simulink model "SVPWM_self"  (R2022a)
settings: Solver=FixedStepAuto  StartTime=0.0  StopTime=stoptime  FixedStep=stepsize  MaxStep=2e-6  RelTol=1e-3
undefined symbols (not defined in the file or in its folder): Continuous, frequency, fs, gcbh, L, R, sps, sps_rtmsupport, spsSawtoothGeneratorModel, stepsize, u_sampletime, V, Vdc
libraries: spsIGBTDiodeLib x6, spsVoltageMeasurementLib x5, spsSeriesRLCBranchLib x4, spsParallelRLCBranchLib x2, spsGroundLib x1, spsThreePhaseVIMeasurementLib x1, spsDCVoltageSourceLib x1, simulink_extras x1, eeTransforms x1, spspowerguiLib x1
settings Model: Creator=Bob  LastModifiedBy=Bob

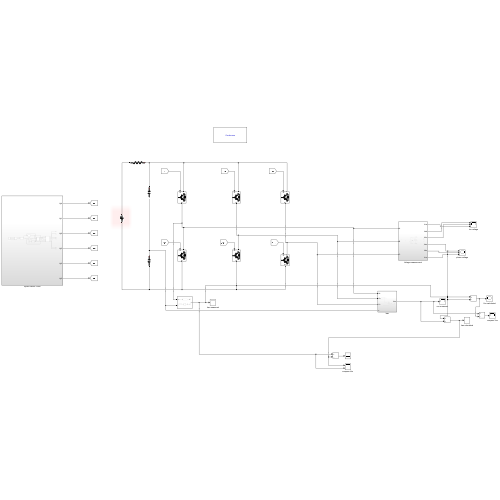
[thumbnail: Simulink's stored preview of the top-level diagram]
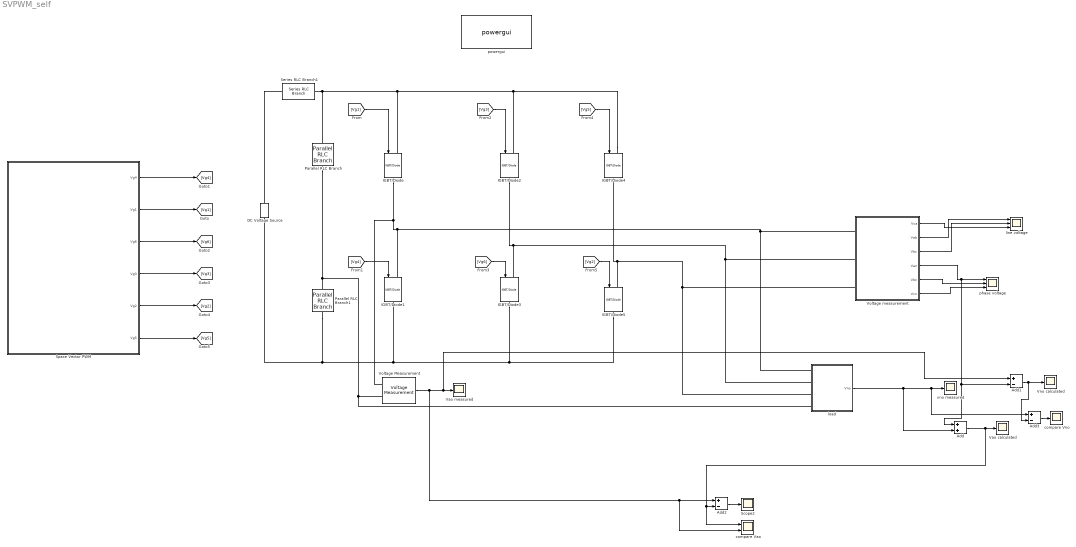
== system SVPWM_self ==
  " load" : Subsystem
  Add : Sum
  Add1 : Sum  Inputs=+-
  Add2 : Sum  Inputs=+-
  Add3 : Sum  Inputs=+-
  DC Voltage Source : spsDCVoltageSourceLib/DC Voltage Source  Amplitude=Vdc  Measurements=None
  IGBT/Diode{,1..5} (6 alike) : spsIGBTDiodeLib/IGBT//Diode  Ron=1e-3  Rs=1e5  Cs=inf  Measurements=off
  Parallel RLC Branch : spsParallelRLCBranchLib/Parallel RLC Branch  LConnTagsString=a  RConnTagsString=__new0  BranchType=C  Resistance=1  Inductance=1e-3  SetiL0=off  InitialCurrent=0  Capacitance=470e-4  Setx0=off  InitialVoltage=1  Measurements=None
  Parallel RLC Branch1 : spsParallelRLCBranchLib/Parallel RLC Branch  LConnTagsString=a  RConnTagsString=__new0  BranchType=C  Resistance=1  Inductance=1e-3  SetiL0=off  InitialCurrent=0  Capacitance=470e-4  Setx0=off  InitialVoltage=1  Measurements=None
  Scope2 : Scope
  Series RLC Branch1 : spsSeriesRLCBranchLib/Series RLC Branch  LConnTagsString=__new0  RConnTagsString=__new0  BranchType=R  Resistance=0.001  Inductance=100e-3  SetiL0=off  InitialCurrent=0  Capacitance=1e-6  Setx0=off  InitialVoltage=0  Measurements=None
  Space Vector PWM : Subsystem
  Vao calculated : Scope
  Vao measured : Scope
  Vno calculated : Scope
  Voltage Measurement : spsVoltageMeasurementLib/Voltage Measurement  PhasorSimulation=off  OutputType=Complex  PSBequivalent=0
  "Voltage measurement " : Subsystem
  compare Vao : Scope  NumInputPorts=2
  compare Vno : Scope
  line voltage : Scope  NumInputPorts=3
  phase voltage : Scope  NumInputPorts=3
  powergui : spspowerguiLib/powergui  Priority=1  SimulationMode=Continuous  SampleTime=stepsize  frequency=60  Iterations=50  frequencyindice=0  Pbase=100e6  ErrMax=1e-4  UnitsV=kV  UnitsW=MW  buscounter=0  FunctionMessages=off  echomessages=off  EnableUseOfTLC=off  CurrentSourceSwitches=off  DisableSnubberDevices=off  DisableRonSwitches=off  DisableVfSwitches=off  DisplayEquations=off  AutomaticDiscreteSolvers=off  SolverType=Tustin/Backward Euler (TBE)  Interpol=off  ExternalGateDelay=off  methode=off  Ts=100  x0status=blocks  SPID=on  SwTol=0  HookPort=off  NonlinearTolerance=1e-4  nMaxIteration=100  ContinueOnMaxIteration=off  RestoreLinks=warning  ResistiveCurrentMeasurement=off  Frange=[0:2:500]  Ylog=off  Xlog=on  ShowGrid=off  save=off  variable=ZData  structure=0  ZoomFFT=off  StartTime=0.0  cycles=1  DisplayStyle=1  fundamental=60  FreqAxis=off  MaxFrequency=1000  frequencyindicesteady=1  RmsSteady=1  display=off
  vno measured : Scope
  wires:
  Space Vector PWM/2(Vg1) -> [Vg1]
  Space Vector PWM/1(Vg4) -> [Vg4]
  Space Vector PWM/3(Vg6) -> [Vg6]
  Space Vector PWM/4(Vg3) -> [Vg3]
  Space Vector PWM/5(Vg2) -> [Vg2]
  Space Vector PWM/6(Vg5) -> [Vg5]
  [Vg6] -> IGBT/Diode3/1
  [Vg2] -> IGBT/Diode5/1
  [Vg3] -> IGBT/Diode2/1
  [Vg4] -> IGBT/Diode1/1
  "Voltage measurement "/1(Vca) -> line voltage/3
  "Voltage measurement "/2(Vab) -> line voltage/1
  "Voltage measurement "/3(Vbc) -> line voltage/2
  "Voltage measurement "/4(Van) -> Add1/2, Add/1, phase voltage/1
  "Voltage measurement "/5(Vbn) -> phase voltage/2
  "Voltage measurement "/6(Vcn) -> phase voltage/3
  [Vg1] -> IGBT/Diode/1
  [Vg5] -> IGBT/Diode4/1
  Voltage Measurement/1 -> compare Vao/2, Add2/1, Add1/1, Vao measured/1
  " load"/1(Vno) -> Add/2, vno measured/1, Add3/1
  Add/1 -> compare Vao/1, Add2/2, Vao calculated/1
  Add1/1 -> Add3/2, Vno calculated/1
  Add2/1 -> Scope2/1
  Add3/1 -> compare Vno/1
  connections:
  IGBT/Diode4/LConn1 -- Parallel RLC Branch/LConn1 -- Series RLC Branch1/LConn1 -- IGBT/Diode/LConn1 -- IGBT/Diode2/LConn1
  IGBT/Diode3/RConn1 -- IGBT/Diode5/RConn1 -- IGBT/Diode1/RConn1 -- Parallel RLC Branch1/RConn1 -- DC Voltage Source/LConn1
  " load"/LConn2 -- "Voltage measurement "/LConn2 -- IGBT/Diode3/LConn1 -- IGBT/Diode2/RConn1
  " load"/LConn1 -- "Voltage measurement "/LConn1 -- IGBT/Diode1/LConn1 -- IGBT/Diode/RConn1 -- Voltage Measurement/LConn1
  " load"/LConn3 -- "Voltage measurement "/LConn3 -- IGBT/Diode4/RConn1 -- IGBT/Diode5/LConn1
  DC Voltage Source/RConn1 -- Series RLC Branch1/RConn1
  Parallel RLC Branch/RConn1 -- " load"/LConn4 -- Voltage Measurement/LConn2 -- Parallel RLC Branch1/LConn1

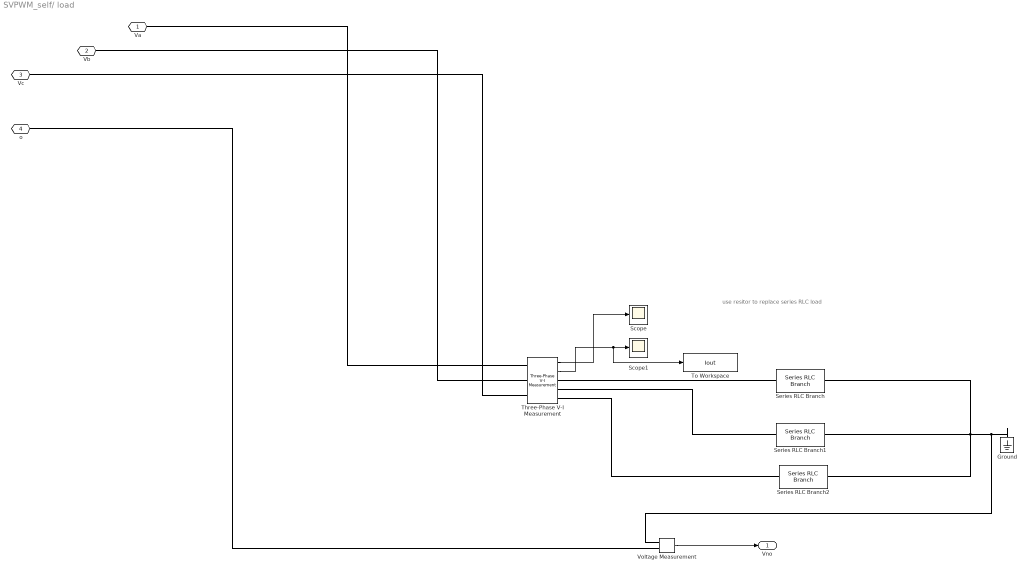
== system SVPWM_self/ load ==
  note: use resitor to replace series RLC load
  Ground : spsGroundLib/Ground  LConnTagsString=a
  Scope : Scope
  Scope1 : Scope
  Series RLC Branch : spsSeriesRLCBranchLib/Series RLC Branch  LConnTagsString=__new0  RConnTagsString=__new0  BranchType=RL  Resistance=R  Inductance=L  SetiL0=off  InitialCurrent=0  Capacitance=1e-6  Setx0=off  InitialVoltage=0  Measurements=None
  Series RLC Branch1 : spsSeriesRLCBranchLib/Series RLC Branch  LConnTagsString=__new0  RConnTagsString=__new0  BranchType=RL  Resistance=R  Inductance=L  SetiL0=off  InitialCurrent=0  Capacitance=1e-6  Setx0=off  InitialVoltage=0  Measurements=None
  Series RLC Branch2 : spsSeriesRLCBranchLib/Series RLC Branch  LConnTagsString=__new0  RConnTagsString=__new0  BranchType=RL  Resistance=R  Inductance=L  SetiL0=off  InitialCurrent=0  Capacitance=1e-6  Setx0=off  InitialVoltage=0  Measurements=None
  Three-Phase V-I Measurement : spsThreePhaseVIMeasurementLib/Three-Phase V-I Measurement  VoltageMeasurement=phase-to-ground  SetLabelV=off  LabelV=Vabc  Vpu=off  VpuLL=off  CurrentMeasurement=yes  SetLabelI=off  LabelI=Iabc  Ipu=off  Pbase=100e6  Vbase=500e3  OutputType=Complex  PhasorSimulation=off  PSBequivalent=0
  To Workspace : ToWorkspace  VariableName=Iout  SampleTime=-1
      settings: Save2DSignal=2-D array (concatenate along first dimension)
  Voltage Measurement : spsVoltageMeasurementLib/Voltage Measurement  PhasorSimulation=off  OutputType=Complex  PSBequivalent=0
  Va : PMIOPort  Side=Left
  Vb : PMIOPort  Port=2  Side=Left
  Vc : PMIOPort  Port=3  Side=Left
  o : PMIOPort  Port=4  Side=Left
  Vno : Outport
  wires:
  Three-Phase V-I Measurement/2 -> To Workspace/1, Scope1/1
  Three-Phase V-I Measurement/1 -> Scope/1
  Voltage Measurement/1 -> Vno/1
  connections:
  Three-Phase V-I Measurement/LConn2 -- Vb/RConn1
  Three-Phase V-I Measurement/LConn3 -- Vc/RConn1
  Three-Phase V-I Measurement/LConn1 -- Va/RConn1
  Ground/LConn1 -- Voltage Measurement/LConn1 -- Series RLC Branch2/RConn1 -- Series RLC Branch1/RConn1 -- Series RLC Branch/RConn1
  Series RLC Branch/LConn1 -- Three-Phase V-I Measurement/RConn1
  Series RLC Branch1/LConn1 -- Three-Phase V-I Measurement/RConn2
  Series RLC Branch2/LConn1 -- Three-Phase V-I Measurement/RConn3
  Voltage Measurement/LConn2 -- o/RConn1

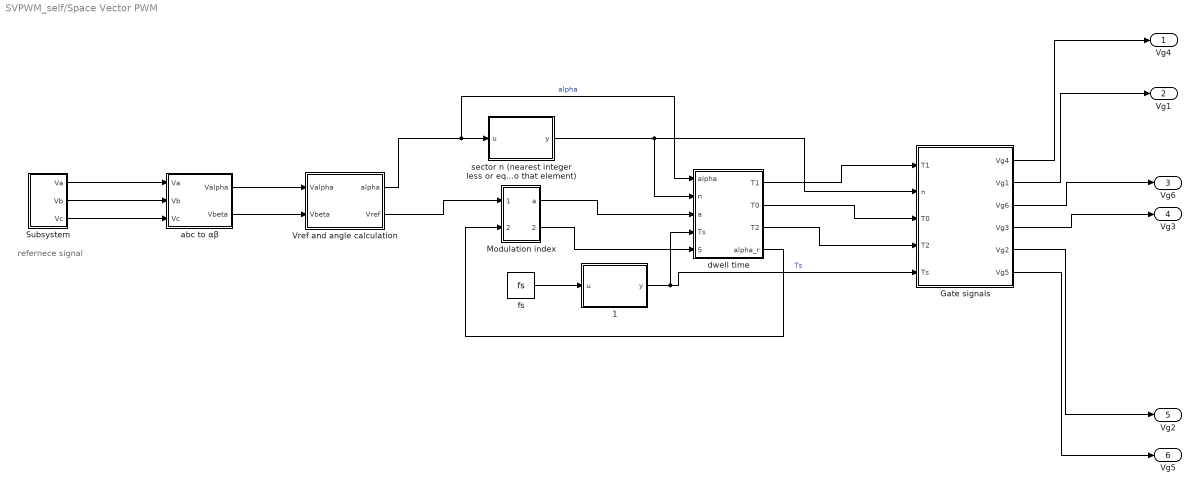
== system SVPWM_self/Space Vector PWM ==
  note: refernece signal
  1 : MATLAB Function  TreatAsAtomicUnit=on
  Gate signals : Subsystem
  Modulation index : Subsystem
  Subsystem : Subsystem
  Vref and angle calculation : Subsystem
  abc to αβ : Subsystem
  "dwell time " : Subsystem
  fs : Constant  Value=fs
  sector n (nearest integer less or equal to that element) : MATLAB Function  TreatAsAtomicUnit=on
  Vg4 : Outport
  Vg1 : Outport  Port=2
  Vg6 : Outport  Port=3
  Vg3 : Outport  Port=4
  Vg2 : Outport  Port=5
  Vg5 : Outport  Port=6
  wires:
  "dwell time "/1(T1) -> Gate signals/1(T1)
  Subsystem/2(Vb) -> abc to αβ/2(Vb)
  Subsystem/3(Vc) -> abc to αβ/3(Vc)
  Vref and angle calculation/1(alpha) -> "dwell time "/1(alpha), sector n (nearest integer less or equal to that element)/1(u)  "alpha"
  abc to αβ/1(Valpha) -> Vref and angle calculation/1(Valpha)
  abc to αβ/2(Vbeta) -> Vref and angle calculation/2(Vbeta)
  Subsystem/1(Va) -> abc to αβ/1(Va)
  Gate signals/2(Vg1) -> Vg1/1
  Vref and angle calculation/2(Vref) -> Modulation index/1(Vref)
  sector n (nearest integer less or equal to that element)/1(y) -> "dwell time "/2(n), Gate signals/2(n)
  "dwell time "/3(T2) -> Gate signals/4(T2)
  Gate signals/5(Vg2) -> Vg2/1
  "dwell time "/2(T0) -> Gate signals/3(T0)
  Gate signals/4(Vg3) -> Vg3/1
  Gate signals/1(Vg4) -> Vg4/1
  Gate signals/3(Vg6) -> Vg6/1
  Gate signals/6(Vg5) -> Vg5/1
  Modulation index/1(a) -> "dwell time "/3(a)
  fs/1 -> 1/1(u)
  1/1(y) -> Gate signals/5(Ts), "dwell time "/4(Ts)  "Ts"
  "dwell time "/4(alpha_r) -> Modulation index/2(alpha_r)
  Modulation index/2(Outport) -> "dwell time "/5(alpha_m)

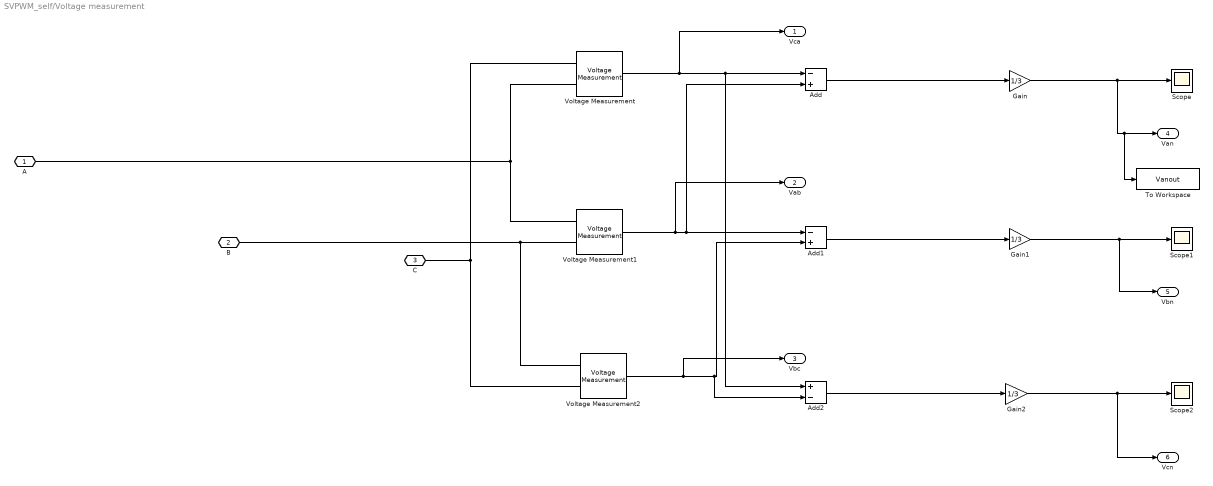
== system SVPWM_self/Voltage measurement  ==
  Add : Sum  Inputs=-+
  Add1 : Sum  Inputs=-+
  Add2 : Sum  Inputs=+-
  Gain : Gain  Gain=1/3
  Gain1 : Gain  Gain=1/3
  Gain2 : Gain  Gain=1/3
  Scope : Scope
  Scope1 : Scope
  Scope2 : Scope
  To Workspace : ToWorkspace  VariableName=Vanout  SampleTime=-1
      settings: Save2DSignal=2-D array (concatenate along first dimension)
  Voltage Measurement : spsVoltageMeasurementLib/Voltage Measurement  PhasorSimulation=off  OutputType=Complex  PSBequivalent=0
  Voltage Measurement1 : spsVoltageMeasurementLib/Voltage Measurement  PhasorSimulation=off  OutputType=Complex  PSBequivalent=0
  Voltage Measurement2 : spsVoltageMeasurementLib/Voltage Measurement  PhasorSimulation=off  OutputType=Complex  PSBequivalent=0
  A : PMIOPort  Side=Left
  B : PMIOPort  Port=2  Side=Left
  C : PMIOPort  Port=3  Side=Left
  Vca : Outport
  Vab : Outport  Port=2
  Vbc : Outport  Port=3
  Van : Outport  Port=4
  Vbn : Outport  Port=5
  Vcn : Outport  Port=6
  wires:
  Gain2/1 -> Vcn/1, Scope2/1
  Gain/1 -> To Workspace/1, Van/1, Scope/1
  Voltage Measurement1/1 -> Vab/1, Add/2, Add1/1
  Voltage Measurement2/1 -> Vbc/1, Add2/2, Add1/2
  Gain1/1 -> Vbn/1, Scope1/1
  Add/1 -> Gain/1
  Add1/1 -> Gain1/1
  Voltage Measurement/1 -> Vca/1, Add2/1, Add/1
  Add2/1 -> Gain2/1
  connections:
  Voltage Measurement/LConn2 -- Voltage Measurement1/LConn1 -- A/RConn1
  Voltage Measurement1/LConn2 -- B/RConn1 -- Voltage Measurement2/LConn1
  Voltage Measurement2/LConn2 -- Voltage Measurement/LConn1 -- C/RConn1

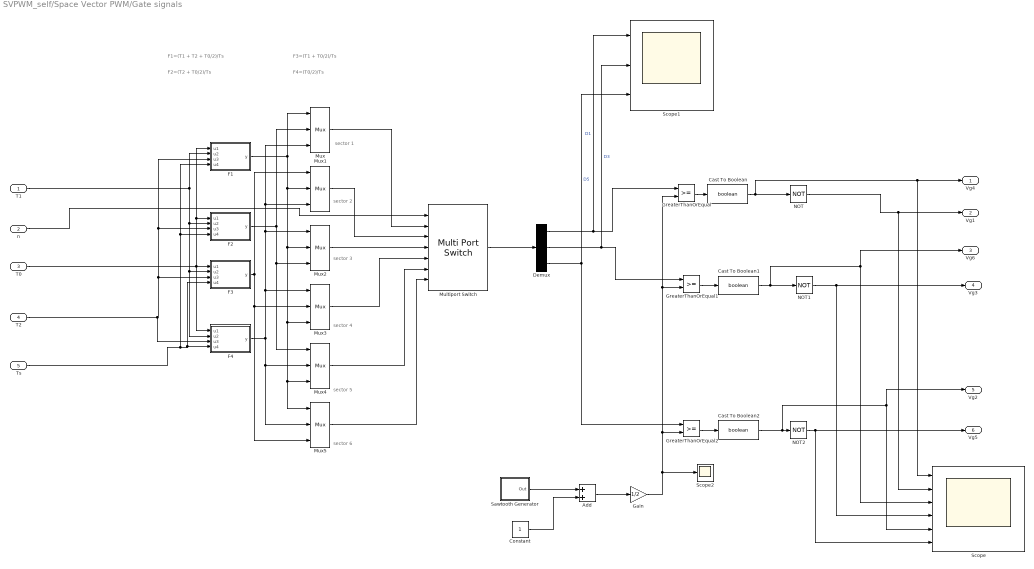
== system SVPWM_self/Space Vector PWM/Gate signals ==
  note: F4=(T0/2)/Ts
  note: F3=(T1 + T0/2)/Ts
  note: F2=(T2 + T0/2)/Ts
  note: F1=(T1 + T2 + T0/2)/Ts
  note: sector 2
  note: sector 3
  note: sector 4
  note: sector 5
  note: sector 6
  note: sector 1
  T1 : Inport
  n : Inport  Port=2
  T0 : Inport  Port=3
  T2 : Inport  Port=4
  Ts : Inport  Port=5
  Add : Sum
  Cast To Boolean : DataTypeConversion  OutDataTypeStr=boolean  SaturateOnIntegerOverflow=off  RndMeth=Floor
  Cast To Boolean1 : DataTypeConversion  OutDataTypeStr=boolean  SaturateOnIntegerOverflow=off  RndMeth=Floor
  Cast To Boolean2 : DataTypeConversion  OutDataTypeStr=boolean  SaturateOnIntegerOverflow=off  RndMeth=Floor
  Constant : Constant
  Demux : Demux  Outputs=3
  F1 : MATLAB Function  TreatAsAtomicUnit=on
  F2 : MATLAB Function  TreatAsAtomicUnit=on
  F3 : MATLAB Function  TreatAsAtomicUnit=on
  F4 : MATLAB Function  TreatAsAtomicUnit=on
  Gain : Gain  Gain=1/2
  GreaterThanOrEqual : RelationalOperator  OutDataTypeStr=boolean  RndMeth=Simplest  InputSameDT=off
  GreaterThanOrEqual1 : RelationalOperator  OutDataTypeStr=boolean  RndMeth=Simplest  InputSameDT=off
  GreaterThanOrEqual2 : RelationalOperator  OutDataTypeStr=boolean  RndMeth=Simplest  InputSameDT=off
  Multiport Switch : MultiPortSwitch  Inputs=6  DiagnosticForDefault=None  SaturateOnIntegerOverflow=off  InputSameDT=off
  Mux{,1..5} (6 alike) : Mux  Inputs=3
  NOT : Logic  Operator=NOT  IconShape=distinctive  AllPortsSameDT=off  OutDataTypeStr=boolean
  NOT1 : Logic  Operator=NOT  IconShape=distinctive  AllPortsSameDT=off  OutDataTypeStr=boolean
  NOT2 : Logic  Operator=NOT  IconShape=distinctive  AllPortsSameDT=off  OutDataTypeStr=boolean
  Sawtooth Generator : Subsystem  AncestorBlock=spsSawtoothGeneratorLib/Sawtooth Generator  DialogController=POWERSYS.PowerSysDialog  LoadFcn=sps_rtmsupport('LoadFcn', gcbh);  StartFcn=sps_rtmsupport('StartFcn', gcbh);  StopFcn=sps_rtmsupport('StopFcn', gcbh);  mask(Sawtooth Generator){Freq=fs, Phase=0, Ts=0}
      mask prompts: Freq "Frequency (Hz):"; Phase "Phase (degrees):"; Ts "Sample time:"
      mask help: Generate a sawtooth wave with peak of -1 to +1.
      mask init:
      | block = gcb;
      | [WantBlockChoice,Ts,sps] = powericon('SawtoothGeneratorInit',block,Phase,Freq,Ts);
      | powericon('SetInternalModels','set',block,WantBlockChoice);
      settings: CopyFcn=sps_rtmsupport('CopyFcn', gcbh);  DeleteFcn=sps_rtmsupport('DeleteFcn', gcbh);  UndoDeleteFcn=sps_rtmsupport('UndoDeleteFcn', gcbh);  ModelCloseFcn=sps_rtmsupport('ModelCloseFcn', gcbh);  PreSaveFcn=sps_rtmsupport('PreSaveFcn', gcbh);  PostSaveFcn=sps_rtmsupport('PostSaveFcn', gcbh);  NameChangeFcn=sps_rtmsupport('NameChangeFcn', gcbh);  PreCopyFcn=sps_rtmsupport('PreCopyFcn', gcbh);  OpenFcn=sps_rtmsupport('OpenFcn', gcbh, []);  CloseFcn=sps_rtmsupport('CloseFcn', gcbh);  PreDeleteFcn=sps_rtmsupport('PreDeleteFcn', gcbh);
      mask Help: helpview(psbhelp);
      mask Display: plot([sps.time sps.time+sps.time(end)],repmat(sps.Out,1,2))
  Scope : Scope  NumInputPorts=6
  Scope1 : Scope  NumInputPorts=3
  Scope2 : Scope
  Vg4 : Outport
  Vg1 : Outport  Port=2
  Vg6 : Outport  Port=3
  Vg3 : Outport  Port=4
  Vg2 : Outport  Port=5
  Vg5 : Outport  Port=6
  wires:
  T0/1 -> F4/1(u1), F1/1(u1), F2/1(u1), F3/1(u1)
  Demux/2 -> Scope1/2, GreaterThanOrEqual1/1  "D3"
  T1/1 -> F4/2(u2), F3/2(u2), F2/2(u2), F1/2(u2)
  n/1 -> Multiport Switch/1
  Gain/1 -> Scope2/1, GreaterThanOrEqual2/2, GreaterThanOrEqual/2, GreaterThanOrEqual1/2
  F1/1(y) -> Mux5/1, Mux4/3, Mux3/3, Mux2/2, Mux1/2, Mux/1
  F4/1(y) -> Mux3/1, Mux2/1, Mux1/3, Mux/3, Mux5/2, Mux4/2
  GreaterThanOrEqual1/1 -> Cast To Boolean1/1
  Mux1/1 -> Multiport Switch/3
  Mux2/1 -> Multiport Switch/4
  NOT1/1 -> Vg3/1, Scope/4
  NOT2/1 -> Vg5/1, Scope/6
  GreaterThanOrEqual/1 -> Cast To Boolean/1
  T2/1 -> F4/3(u3), F3/3(u3), F2/3(u3), F1/3(u3)
  Mux/1 -> Multiport Switch/2
  GreaterThanOrEqual2/1 -> Cast To Boolean2/1
  NOT/1 -> Vg1/1, Scope/2
  Ts/1 -> F1/4(u4), F2/4(u4), F3/4(u4), F4/4(u4)
  Demux/1 -> Scope1/1, GreaterThanOrEqual/1  "D1"
  Demux/3 -> GreaterThanOrEqual2/1, Scope1/3  "D5"
  F3/1(y) -> Mux1/1, Mux5/3, Mux3/2
  Mux5/1 -> Multiport Switch/7
  Mux3/1 -> Multiport Switch/5
  F2/1(y) -> Mux4/1, Mux2/3, Mux/2
  Sawtooth Generator/1(Out) -> Add/1
  Multiport Switch/1 -> Demux/1
  Mux4/1 -> Multiport Switch/6
  Add/1 -> Gain/1
  Constant/1 -> Add/2
  Cast To Boolean/1 -> Vg4/1, Scope/1, NOT/1
  Cast To Boolean1/1 -> Vg6/1, Scope/3, NOT1/1
  Cast To Boolean2/1 -> Vg2/1, Scope/5, NOT2/1

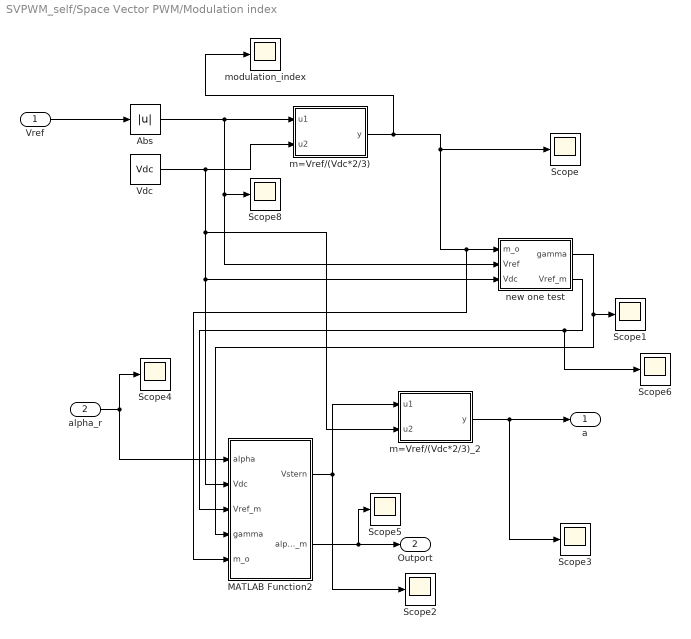
== system SVPWM_self/Space Vector PWM/Modulation index ==
  Vref : Inport
  alpha_r : Inport  Port=2
  Abs : Abs  SaturateOnIntegerOverflow=off
  MATLAB Function2 : MATLAB Function  TreatAsAtomicUnit=on
  Scope{,1..6,8} (8 alike) : Scope
  Vdc : Constant  Value=Vdc
  m=Vref/(Vdc*2/3) : MATLAB Function  TreatAsAtomicUnit=on
  m=Vref/(Vdc*2/3)_2 : MATLAB Function  TreatAsAtomicUnit=on
  modulation_index : Scope
  new one test : MATLAB Function  TreatAsAtomicUnit=on
  a : Outport
  Outport : Outport  Port=2
  wires:
  Abs/1 -> new one test/2(Vref), Scope8/1, m=Vref/(Vdc*2/3)/1(u1)
  m=Vref/(Vdc*2/3)/1(y) -> MATLAB Function2/5(m_o), new one test/1(m_o), Scope/1, modulation_index/1
  Vref/1 -> Abs/1
  Vdc/1 -> m=Vref/(Vdc*2/3)/2(u2), new one test/3(Vdc), MATLAB Function2/2(Vdc), m=Vref/(Vdc*2/3)_2/2(u2)
  alpha_r/1 -> MATLAB Function2/1(alpha), Scope4/1
  MATLAB Function2/1(Vstern) -> Scope2/1, m=Vref/(Vdc*2/3)_2/1(u1)
  m=Vref/(Vdc*2/3)_2/1(y) -> Scope3/1, a/1
  new one test/1(gamma) -> Scope1/1, MATLAB Function2/4(gamma)
  MATLAB Function2/2(alpha_m) -> Scope5/1, Outport/1
  new one test/2(Vref_m) -> Scope6/1, MATLAB Function2/3(Vref_m)

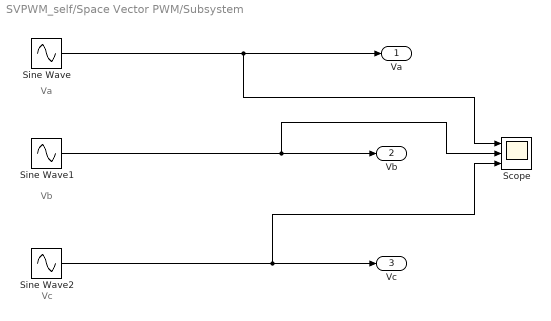
== system SVPWM_self/Space Vector PWM/Subsystem ==
  note: Va
  note: Vb
  note: Vc
  Scope : Scope  NumInputPorts=3
  Sine Wave : Sin  Amplitude=V  Frequency=2*pi*frequency  SampleTime=0
  Sine Wave1 : Sin  Amplitude=V  Frequency=2*pi*frequency  Phase=-2*pi/3  SampleTime=0
  Sine Wave2 : Sin  Amplitude=V  Frequency=2*pi*frequency  Phase=-4*pi/3  SampleTime=0
  Va : Outport
  Vb : Outport  Port=2
  Vc : Outport  Port=3
  wires:
  Sine Wave1/1 -> Vb/1, Scope/2
  Sine Wave2/1 -> Vc/1, Scope/3
  Sine Wave/1 -> Va/1, Scope/1

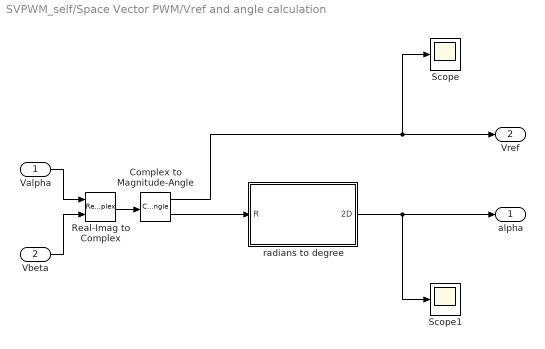
== system SVPWM_self/Space Vector PWM/Vref and angle calculation ==
  Valpha : Inport
  Vbeta : Inport  Port=2
  Complex to Magnitude-Angle : ComplexToMagnitudeAngle
  Real-Imag to Complex : RealImagToComplex
  Scope : Scope
  Scope1 : Scope
  radians to degree : Subsystem
  alpha : Outport
  Vref : Outport  Port=2
  wires:
  Complex to Magnitude-Angle/2 -> radians to degree/1(R)
  Complex to Magnitude-Angle/1 -> Scope/1, Vref/1
  Valpha/1 -> Real-Imag to Complex/1
  Vbeta/1 -> Real-Imag to Complex/2
  radians to degree/1(2D) -> Scope1/1, alpha/1
  Real-Imag to Complex/1 -> Complex to Magnitude-Angle/1

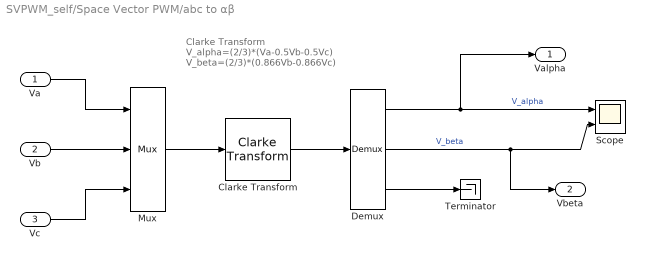
== system SVPWM_self/Space Vector PWM/abc to αβ ==
  note: Clarke Transform
      | V_alpha=(2/3)*(Va-0.5Vb-0.5Vc)
      | V_beta=(2/3)*(0.866Vb-0.866Vc)
  Va : Inport
  Vb : Inport  Port=2
  Vc : Inport  Port=3
  Clarke Transform : eeTransforms/Clarke Transform  PowerInvariant=off
      settings: SourceProductBaseCode=PS
  Demux : Demux  Outputs=3
  Mux : Mux  Inputs=3
  Scope : Scope  NumInputPorts=2
  Terminator : Terminator
  Valpha : Outport
  Vbeta : Outport  Port=2
  wires:
  Demux/2 -> Vbeta/1, Scope/2  "V_beta"
  Clarke Transform/1 -> Demux/1
  Demux/3 -> Terminator/1
  Demux/1 -> Valpha/1, Scope/1  "V_alpha"
  Va/1 -> Mux/1
  Vb/1 -> Mux/2
  Vc/1 -> Mux/3
  Mux/1 -> Clarke Transform/1

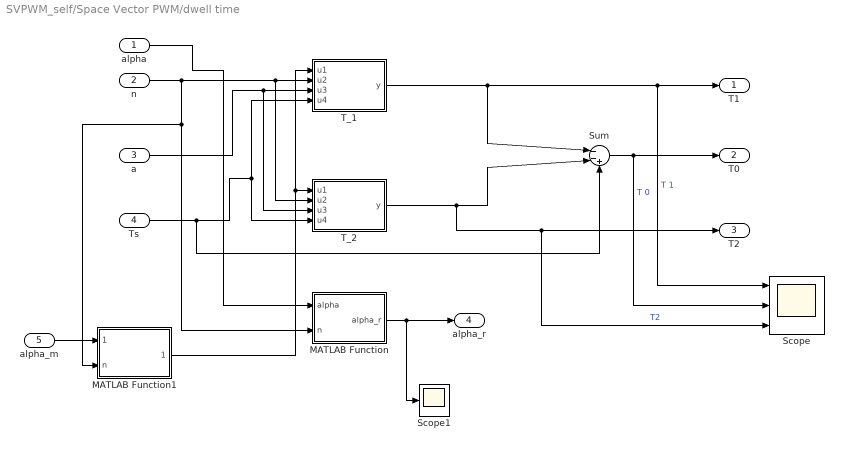
== system SVPWM_self/Space Vector PWM/dwell time  ==
  alpha : Inport
  n : Inport  Port=2
  a : Inport  Port=3
  Ts : Inport  Port=4
  alpha_m : Inport  Port=5
  MATLAB Function : MATLAB Function  TreatAsAtomicUnit=on
  MATLAB Function1 : MATLAB Function  TreatAsAtomicUnit=on
  Scope : Scope  NumInputPorts=3
  Scope1 : Scope
  Sum : Sum  Inputs=|--+
  T_1 : MATLAB Function  TreatAsAtomicUnit=on
  T_2 : MATLAB Function  TreatAsAtomicUnit=on
  T1 : Outport
  T0 : Outport  Port=2
  T2 : Outport  Port=3
  alpha_r : Outport  Port=4
  wires:
  T_1/1(y) -> Scope/1, T1/1, Sum/1  "T 1"
  T_2/1(y) -> Scope/3, T2/1, Sum/2  "T2"
  alpha/1 -> MATLAB Function/1(alpha)
  n/1 -> MATLAB Function1/2(n), MATLAB Function/2(n), T_2/2(u2), T_1/2(u2)
  a/1 -> T_2/3(u3), T_1/3(u3)
  Ts/1 -> Sum/3, T_1/4(u4), T_2/4(u4)
  Sum/1 -> Scope/2, T0/1  "T 0"
  MATLAB Function/1(alpha_r) -> Scope1/1, alpha_r/1
  alpha_m/1 -> MATLAB Function1/1(alpha_m)
  MATLAB Function1/1(alpha_mr) -> T_2/1(u1), T_1/1(u1)

== system SVPWM_self/Space Vector PWM/Gate signals/Sawtooth Generator ==
  Model : Subsystem  AncestorBlock=spsSawtoothGeneratorModel/Continuous
  Out : Outport  VectorParamsAs1DForOutWhenUnconnected=off
  wires:
  Model/1(Out) -> Out/1

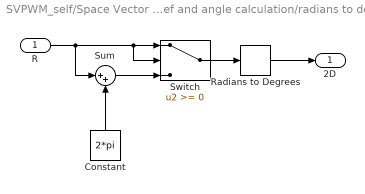
== system SVPWM_self/Space Vector PWM/Vref and angle calculation/radians to degree ==
  R : Inport
  Constant : Constant  Value=2*pi
  Radians to Degrees : simulink_extras/Transformations/Radians to Degrees
  Sum : Sum  Inputs=|++
  Switch : Switch  SaturateOnIntegerOverflow=off  InputSameDT=off
  2D : Outport
  wires:
  Radians to Degrees/1 -> 2D/1
  Constant/1 -> Sum/2
  R/1 -> Sum/1, Switch/2, Switch/1
  Sum/1 -> Switch/3
  Switch/1 -> Radians to Degrees/1

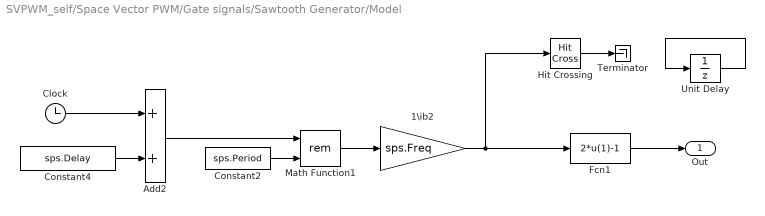
== system SVPWM_self/Space Vector PWM/Gate signals/Sawtooth Generator/Model ==
  1\ib2 : Gain  Gain=sps.Freq  SaturateOnIntegerOverflow=on  OutDataTypeStr=Inherit: Same as input  ParamDataTypeStr=Inherit: Same as input
  Add2 : Sum
  Clock : Clock
  Constant2 : Constant  Value=sps.Period  SampleTime=0
  Constant4 : Constant  Value=sps.Delay  SampleTime=0
  Fcn1 : Fcn  Expr=2*u(1)-1
  Hit Crossing : HitCross
  Math Function1 : Math  Operator=rem  SignedPower=on
  Terminator : Terminator
  Unit Delay : UnitDelay  SampleTime=u_sampletime  HasFrameUpgradeWarning=on
  Out : Outport
  wires:
  Math Function1/1 -> 1\ib2/1
  Clock/1 -> Add2/1
  Constant2/1 -> Math Function1/2
  Constant4/1 -> Add2/2
  Add2/1 -> Math Function1/1
  Unit Delay/1 -> Unit Delay/1
  Fcn1/1 -> Out/1
  1\ib2/1 -> Hit Crossing/1, Fcn1/1
  Hit Crossing/1 -> Terminator/1

== matlab function SVPWM_self/Space Vector PWM/dwell time /MATLAB Function1 ==
  data: alpha_m input; alpha_mr output; n input
function alpha_mr = fcn(alpha_m,n)
alpha_mr=(alpha_m*180/pi+((n-1)*(60)));

== matlab function SVPWM_self/Space Vector PWM/Modulation index/m=Vref//(Vdc*2//3)_2 ==
  data: u1 input; y output; u2 input
function y = fcn(u1,u2)

y = u1/((2/3)*u2);

== matlab function SVPWM_self/Space Vector PWM/Modulation index/MATLAB Function2 ==
  data: alpha input; Vstern output; Vdc input; Vref_m input; gamma input; m_o input; alpha_m output
function [Vstern,alpha_m] = fcn(alpha,Vdc,Vref_m,gamma,m_o)
Vstern=0;
alpha_m=pi;
if gamma==pi/2
    Vstern=Vref_m;
    alpha_m=alpha;
end
if gamma~=pi/2
    if ((m_o>(sqrt(3)/2))&&(m_o<0.9068))
        if ((0<=alpha)&&(alpha<(gamma)))
            Vstern=Vref_m;
            alpha_m=alpha;
        end
        if ((alpha>=(gamma))&&(alpha<((pi/3)-gamma)))
            if (alpha<=(pi/6))
                Vstern=(1/sqrt(3))*Vdc/(cos((pi/6)-alpha)) ;
                alpha_m=alpha;
            end
            if (alpha>(pi/6))
                Vstern=(1/sqrt(3))*Vdc/(cos(alpha-(pi/6))) ;
                alpha_m=alpha;
            end
        end
        if ((((pi/3)-gamma)<=alpha)&&(alpha<(pi/3)))
            Vstern=Vref_m;
            alpha_m=alpha;
        end
    end
    if ((m_o>=0.9068)&&(m_o<0.9517))
        if ((0<=alpha)&&(alpha<(gamma)))
            Vstern=(1/sqrt(3))*Vdc/(cos((pi/6)-alpha));
            alpha_m=alpha;
        end
        if ((alpha>=(gamma))&&(alpha<((pi/3)-gamma)))
            if (alpha<=(pi/6))
                Vstern=(1/sqrt(3))*Vdc/(cos((pi/6)-alpha)) ;
                alpha_m=alpha;
            end
            if (alpha>(pi/6))
                Vstern=(1/sqrt(3))*Vdc/(cos(alpha-(pi/6))) ;
                alpha_m=alpha;
            end
        end
        if ((((pi/3)-gamma)<=alpha)&&(alpha<(pi/3)))
            Vstern=(1/sqrt(3))*Vdc/(cos(alpha-(pi/6))) ;
            alpha_m=alpha;
        end
    end
    if (m_o>=0.9517)
        if ((0<=alpha)&&(alpha<(gamma)))
            Vstern=2*Vdc/3;
            alpha_m=0;
        end
        if ((alpha>=(gamma))&&(alpha<((pi/3)-gamma)))
            if (alpha<=(pi/6))
                Vstern=(1/sqrt(3))*Vdc/(cos((pi/6)-alpha)) ;
                alpha_m=(pi/6)*(alpha-gamma)/((pi/6)-gamma);
            end
            if (alpha>(pi/6))
                Vstern=(1/sqrt(3))*Vdc/(cos(alpha-(pi/6))) ;
                alpha_m=(pi/6)+(pi/6)*(alpha-(pi/6))/((pi/6)-gamma);
            end
        end
        if ((((pi/3)-gamma)<=alpha)&&(alpha<(pi/3)))
            Vstern=2*Vdc/3;
            alpha_m=pi/3;
        end
    end
end
%  if ((alpha>=((pi/3)-gamma))&&(alpha<=(pi/3)))
%      if ((pi/3)-gamma)<0
%         Vstern=Vref;
%      end
%         if ((pi/3)-gamma)>=0
%             Vstern=(1/sqrt(3))*Vdc*1/(cos((pi/6)-gamma));
%         end
%  end
%
%
%

== matlab function SVPWM_self/Space Vector PWM/dwell time /MATLAB Function ==
  data: alpha input; alpha_r output; n input
function alpha_r = fcn(alpha,n)
alpha_r=(alpha*pi/180-((n-1)*(pi/3)));

== matlab function SVPWM_self/Space Vector PWM/sector n (nearest integer less or equal to that element) ==
  data: u input; y output
function y = fcn(u)

y = floor(u/60)+1;

== matlab function SVPWM_self/Space Vector PWM/Modulation index/m=Vref//(Vdc*2//3) ==
  data: u1 input; y output; u2 input
function y = fcn(u1,u2)

y = u1/((2/3)*u2);

== matlab function SVPWM_self/Space Vector PWM/dwell time /T_1 ==
  data: u1 input; y output; u2 input; u3 input; u4 input
function y = fcn(u1,u2,u3,u4)

y =[u3*u4*sin(u2*pi/3-u1*pi/180)]/sin(pi/3);

== matlab function SVPWM_self/Space Vector PWM/dwell time /T_2 ==
  data: u1 input; y output; u2 input; u3 input; u4 input
function y = fcn(u1,u2,u3,u4)

y =[u3*u4*sin(u1*pi/180-(u2-1)*pi/3)]/sin(pi/3);

== matlab function SVPWM_self/Space Vector PWM/Gate signals/F1 ==
  data: u1 input; y output; u2 input; u3 input; u4 input
function y = fcn(u1,u2,u3,u4)

y = (u2+u3+u1/2)/u4;

== matlab function SVPWM_self/Space Vector PWM/Gate signals/F2 ==
  data: u1 input; y output; u2 input; u3 input; u4 input
function y = fcn(u1,u2,u3,u4)

y = (u3+u1/2)/u4;

== matlab function SVPWM_self/Space Vector PWM/Gate signals/F3 ==
  data: u1 input; y output; u2 input; u3 input; u4 input
function y = fcn(u1,u2,u3,u4)

y = (u2+u1/2)/u4;

== matlab function SVPWM_self/Space Vector PWM/Gate signals/F4 ==
  data: u1 input; y output; u2 input; u3 input; u4 input
function y = fcn(u1,u2,u3,u4)

y = (u1/2)/u4;

== matlab function SVPWM_self/Space Vector PWM/1 ==
  data: u input; y output
function y = fcn(u)

y = 1/u;

== matlab function SVPWM_self/Space Vector PWM/Modulation index/new one test ==
  data: m_o input; gamma output; Vref input; Vdc input; Vref_m output
function [gamma,Vref_m]= fcn(m_o,Vref,Vdc)
gamma=pi/2;
Vref_m=0;
if (m_o<=(sqrt(3)/2))
    gamma=pi/2;
    Vref_m=Vref;
end
if ((m_o>(sqrt(3)/2))&&(m_o<0.9068))

    x=linspace(Vdc/3,Vdc*2/3,1e4);
    y1=(-sqrt(3)).*x+(2*Vdc/sqrt(3));
    % for n11=1:1e5
    y2= y1.^2+x.^2-Vref^2;
    [~,idx]=min(abs(y2));
    minVal=y1(idx);
    gamma1=atan((minVal)/(x(idx)));
    if gamma1<(pi/6)
        gamma=gamma1;
        Vref_m=Vref;
    end
    if gamma1>=(pi/6)
        gamma=(pi/3)-gamma1;
        Vref_m=Vref;
    end
end
if ((m_o>=0.9068)&&(m_o<=0.9095))
    gamma=-30.23.*m_o+27.94;
    Vref_m=Vref;
end
if ((m_o>=0.9095)&&(m_o<0.9485))
    gamma=-8.58.*m_o+8.23;
    Vref_m=Vref;
end
if ((m_o>=0.9485)&&(m_o<0.9517))
    gamma=-26.43.*m_o+25.15;
    Vref_m=Vref;
end
if ((m_o>=0.9517)&&(m_o<0.98))
    gamma=6.4.*m_o-6.09;
    Vref_m=Vref;
end
if ((m_o>=0.98)&&(m_o<0.9975))
    gamma=11.75.*m_o-11.34;
    Vref_m=Vref;
end
if (m_o>=0.9975)
    gamma=48.96.*m_o-48.3;
    Vref_m=Vref;
end
%
% x=[ ((2/3)*Vdc) ((1/3)*Vdc)];
% y=[ 0 ((1/sqrt(3))*Vdc)];
% figure;
% plot(x,y);  ===== ===== 00
% hold;
% th = 0:pi/50:2*pi;
% xunit = Vref * cos(th) ;
% yunit = Vref * sin(th) ;
% plot(xunit, yunit);
% [xi,yi] = polyxpoly(x,y,xunit,yunit);
% gamma=atan((f1)/(xi(1,1)));
% end
